simulink model "VehiclePlant"  (R2026b)
settings: Solver=ode23t  StopTime=Simulation.StopTimeSmoke.Value
undefined symbols (not defined in the file): Battery, Brake, Tire
settings Model: DataDictionary=VehicleData.sldd  Creator=Xu Dingyi  LastModifiedBy=29358
settings DebuggingCC: AlgebraicLoopMsg=error  ArtificialAlgebraicLoopMsg=error  BusObjectLabelMismatch=error

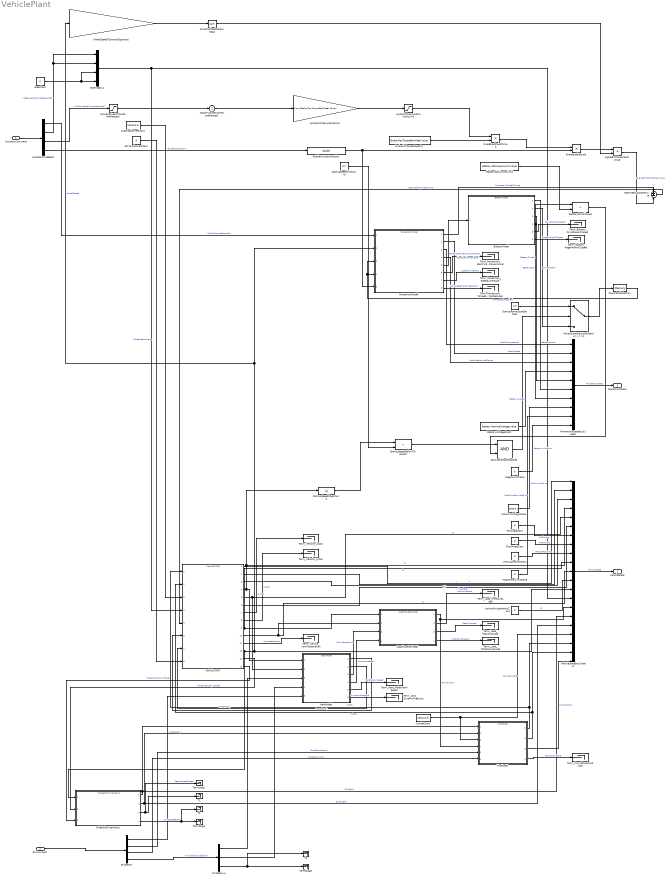
== system VehiclePlant ==
  ActuatorCommand : Inport  OutDataTypeStr=Bus: ActuatorCommandBus
  Environment : Inport  Port=2  OutDataTypeStr=Bus: EnvironmentBus
  ActuatorCmdSelect : BusSelector  OutputSignals=MotorTorqueRequest,SteeringRackAngleRequest,FrictionBrakeTorqueRequest,EnableActuation
  AeroModel : ModelReference  ModelNameDialog=AeroModel.slx  ModelReferenceVersion=2.0
  AligningMomentZero : Constant  Value=zeros(4,1)  OutDataTypeStr=double
  BatteryModel : ModelReference  ModelNameDialog=BatteryModel.slx  ModelReferenceVersion=2.0
  BatterySOCAllowed : RelationalOperator  Operator=>  OutDataTypeStr=boolean  InputSameDT=off
  BatterySOCLowerLimit : Constant  Value=Battery.SOCLowerLimit.Value  OutDataTypeStr=double
  BatteryVoltageConst : Constant  Value=Battery.NominalVoltage.Value  OutDataTypeStr=double
  BrakeEnableScale : Product  Inputs=**
  CamberZero : Constant  Value=zeros(4,1)  OutDataTypeStr=double
  EnableActuationDouble : DataTypeConversion  OutDataTypeStr=double
  EnvSelect : BusSelector  OutputSignals=AirDensity,RoadGripScale,RoadMuLimit,WindVelocityGlobal
  ExtYawMomentZero : Constant  Value=0  OutDataTypeStr=double
  FixedBiasBrakeTorque : Product  Inputs=**
  HydraulicPressureFraction : Gain  Gain=1/sum(Brake.MaxTorquePerWheel.Value)
  HydraulicPressureFractionLimit : Saturate  UpperLimit=1  LowerLimit=0
  HydraulicTorqueCapacity : Constant  Value=Brake.MaxTorquePerWheel.Value
  LoadTransferModel : ModelReference  ModelNameDialog=LoadTransferModel.slx  ModelReferenceVersion=2.1
  MotorLimitFlagsFalse : Constant  Value=false(4,1)  OutDataTypeStr=boolean
  NetWheelAppliedTorque : Sum  Inputs=+-
  NonnegativeFrictionBrakeRequest : Saturate  UpperLimit=inf(4,1)  LowerLimit=zeros(4,1)
  PitchAngleZero : Constant  Value=0  OutDataTypeStr=double
  PowerScaleMemory : Memory  InitialCondition=1
  PowerScaleStartupFallback : Switch  Threshold=0.5
  PowertrainModel : ModelReference  ModelNameDialog=PowertrainModel.slx  ModelReferenceVersion=2.0
  PowertrainStateBusCreator : BusCreator  Inputs=10  OutDataTypeStr=Bus: PowertrainStateBus
  RegenLimitFalse : Constant  Value=0  OutDataTypeStr=boolean
  RollAngleZero : Constant  Value=0  OutDataTypeStr=double
  SignedFrictionBrakeTorque : Product  Inputs=**
  SmoothWheelRotationSign : Trigonometry  Description=Continuous wheel-rotation sign approximation for stable friction braking through zero speed.  Operator=tanh
  StartupFallbackEnabled : Logic  AllPortsSameDT=off  OutDataTypeStr=boolean
  StartupPowerScaleDefault : Constant  Value=1.0  OutDataTypeStr=double
  StartupSpeedBelowThreshold : RelationalOperator  Operator=<  OutDataTypeStr=boolean  InputSameDT=off
  StartupSpeedMagnitude : Abs
  StartupSpeedThreshold : Constant  Value=0.1  OutDataTypeStr=double
  SteerZero : Constant  Value=0  OutDataTypeStr=double
  SteeringMux : Mux
  T1 : Terminator
  T2 : Terminator
  T3 : Terminator
  TermDiag1 : Terminator
  TermDiag2 : Terminator
  TermDiag3 : Terminator
  Term_Aero_DynamicPressure : Terminator
  Term_Aero_RelativeAirSpeed : Terminator
  Term_Battery_DrivePowerClipped : Terminator
  Term_Battery_RegenPowerClipped : Terminator
  Term_Load_FrontAxleLoad : Terminator
  Term_Load_RearAxleLoad : Terminator
  Term_Load_TotalNormalLoad : Terminator
  Term_Powertrain_ElectricalPowerActual : Terminator
  Term_Powertrain_SpeedLimitScale : Terminator
  Term_Powertrain_TorqueSaturationResidual : Terminator
  Term_Tire_SaturationScale : Terminator
  Term_Vehicle_UxDot : Terminator
  Term_Vehicle_UyDot : Terminator
  Term_Vehicle_YawAcceleration : Terminator
  TireModel : ModelReference  ModelNameDialog=TireModel  ModelReferenceVersion=2.0
  TotalFrictionBrakeTorqueRequest : Sum  Inputs=+
  TotalPowerLimitFalse : Constant  Value=0  OutDataTypeStr=boolean
  Vehicle7DOF : ModelReference  ModelNameDialog=Vehicle7DOF.slx  ModelReferenceVersion=2.0
  VehicleStateBusCreator : BusCreator  Inputs=21  OutDataTypeStr=Bus: VehicleStateBus
  VerticalAccelerationZero : Constant  Value=0  OutDataTypeStr=double
  VerticalPositionZero : Constant  Value=0  OutDataTypeStr=double
  WheelSlipKinematics : ModelReference  ModelNameDialog=WheelSlipKinematics.slx  ModelReferenceVersion=2.0
  WheelSpeedToSmoothSignInput : Gain  Gain=Tire.EffectiveRadius.Value/Tire.LowSpeedEpsilon.Value
  WindDemux : Demux  Outputs=3
  VehicleState : Outport  OutDataTypeStr=Bus: VehicleStateBus
  PowertrainState : Outport  Port=2  OutDataTypeStr=Bus: PowertrainStateBus
  wires:
  StartupSpeedThreshold/1 -> StartupSpeedBelowThreshold/2
  SteeringMux/1 -> VehicleStateBusCreator/14, Vehicle7DOF/4  "WheelSteerAngle"
  ActuatorCommand/1 -> ActuatorCmdSelect/1
  ActuatorCmdSelect/2 -> SteeringMux/2, SteeringMux/1  "<SteeringRackAngleRequest>"
  Environment/1 -> EnvSelect/1
  StartupSpeedMagnitude/1 -> StartupSpeedBelowThreshold/1
  SteerZero/1 -> SteeringMux/3, SteeringMux/4
  ActuatorCmdSelect/1 -> PowertrainModel/1  "<MotorTorqueRequest>"
  ActuatorCmdSelect/3 -> NonnegativeFrictionBrakeRequest/1  "<FrictionBrakeTorqueRequest>"
  ActuatorCmdSelect/4 -> EnableActuationDouble/1  "<EnableActuation>"
  TireModel/1 -> Vehicle7DOF/1, VehicleStateBusCreator/19  "TireFx"
  WheelSpeedToSmoothSignInput/1 -> SmoothWheelRotationSign/1
  LoadTransferModel/1 -> TireModel/4, VehicleStateBusCreator/15  "NormalLoad"
  NonnegativeFrictionBrakeRequest/1 -> TotalFrictionBrakeTorqueRequest/1
  AligningMomentZero/1 -> Vehicle7DOF/3
  EnvSelect/1 -> AeroModel/5  "<AirDensity>"
  ExtYawMomentZero/1 -> Vehicle7DOF/8
  StartupPowerScaleDefault/1 -> PowerScaleStartupFallback/1
  WindDemux/3 -> TermDiag3/1, T3/1
  WheelSlipKinematics/1 -> VehicleStateBusCreator/16, TireModel/1  "SlipRatio"
  WheelSlipKinematics/2 -> TireModel/2, VehicleStateBusCreator/17  "SlipAngle"
  WheelSlipKinematics/3 -> TermDiag1/1, T1/1  "RegularizedSpeed"
  WheelSlipKinematics/4 -> T2/1, TermDiag2/1  "LowSpeedBlend"
  EnableActuationDouble/1 -> BrakeEnableScale/2, PowertrainModel/5
  EnvSelect/2 -> TireModel/5  "<RoadGripScale>"
  CamberZero/1 -> VehicleStateBusCreator/18, TireModel/3  "CamberAngle"
  SmoothWheelRotationSign/1 -> SignedFrictionBrakeTorque/2
  TotalFrictionBrakeTorqueRequest/1 -> HydraulicPressureFraction/1
  Vehicle7DOF/13 -> WheelSlipKinematics/2  "WheelVelocityXWheel"
  Vehicle7DOF/9 -> LoadTransferModel/1, VehicleStateBusCreator/10  "Ax"
  Vehicle7DOF/5 -> VehicleStateBusCreator/5, AeroModel/2  "Uy"
  Vehicle7DOF/1 -> VehicleStateBusCreator/1  "X"
  Vehicle7DOF/14 -> WheelSlipKinematics/3  "WheelVelocityYWheel"
  Vehicle7DOF/10 -> VehicleStateBusCreator/11, LoadTransferModel/2  "Ay"
  Vehicle7DOF/6 -> VehicleStateBusCreator/6  "YawRate"
  Vehicle7DOF/2 -> VehicleStateBusCreator/2  "Y"
  Vehicle7DOF/11 -> Term_Vehicle_YawAcceleration/1  "YawAcceleration"
  Vehicle7DOF/7 -> Term_Vehicle_UxDot/1  "UxDot"
  Vehicle7DOF/3 -> VehicleStateBusCreator/3  "Psi"
  Vehicle7DOF/12 -> WheelSpeedToSmoothSignInput/1, PowertrainModel/2, VehicleStateBusCreator/13, WheelSlipKinematics/1  "WheelSpeed"
  Vehicle7DOF/8 -> Term_Vehicle_UyDot/1  "UyDot"
  Vehicle7DOF/4 -> VehicleStateBusCreator/4, StartupSpeedMagnitude/1, AeroModel/1  "Ux"
  WindDemux/1 -> AeroModel/3
  WindDemux/2 -> AeroModel/4
  HydraulicPressureFraction/1 -> HydraulicPressureFractionLimit/1
  AeroModel/1 -> Vehicle7DOF/6  "ForceXBody"
  AeroModel/6 -> Term_Aero_DynamicPressure/1  "DynamicPressure"
  AeroModel/4 -> LoadTransferModel/4  "DownforceRear"
  AeroModel/2 -> Vehicle7DOF/7  "ForceYBody"
  AeroModel/5 -> Term_Aero_RelativeAirSpeed/1  "RelativeAirSpeed"
  AeroModel/3 -> LoadTransferModel/3  "DownforceFront"
  HydraulicPressureFractionLimit/1 -> FixedBiasBrakeTorque/1
  HydraulicTorqueCapacity/1 -> FixedBiasBrakeTorque/2
  PowertrainModel/1 -> NetWheelAppliedTorque/1  "PowertrainWheelTorque"
  PowertrainModel/2 -> PowertrainStateBusCreator/2  "MotorSpeed"
  PowertrainModel/3 -> PowertrainStateBusCreator/1  "MotorTorqueActual"
  PowertrainModel/8 -> Term_Powertrain_TorqueSaturationResidual/1  "TorqueSaturationResidual"
  PowertrainModel/4 -> PowertrainStateBusCreator/3  "MotorMechanicalPower"
  PowertrainModel/5 -> BatteryModel/1  "ElectricalPowerUnconstrained"
  PowertrainModel/6 -> Term_Powertrain_ElectricalPowerActual/1  "ElectricalPowerActual"
  PowertrainModel/7 -> Term_Powertrain_SpeedLimitScale/1  "SpeedLimitScale"
  StartupSpeedBelowThreshold/1 -> StartupFallbackEnabled/1
  LoadTransferModel/2 -> Term_Load_FrontAxleLoad/1  "FrontAxleLoad"
  LoadTransferModel/3 -> Term_Load_RearAxleLoad/1  "RearAxleLoad"
  LoadTransferModel/4 -> Term_Load_TotalNormalLoad/1  "TotalNormalLoad"
  FixedBiasBrakeTorque/1 -> BrakeEnableScale/1
  BatterySOCLowerLimit/1 -> BatterySOCAllowed/2
  BatteryModel/1 -> PowertrainStateBusCreator/6  "BatteryPower"
  BatteryModel/2 -> PowerScaleStartupFallback/3  "PowerScale"
  BatteryModel/3 -> PowertrainStateBusCreator/5  "BatteryCurrent"
  BatteryModel/4 -> BatterySOCAllowed/1, PowertrainStateBusCreator/7  "BatterySOC"
  BatteryModel/5 -> Term_Battery_DrivePowerClipped/1  "DrivePowerClipped"
  BatteryModel/6 -> Term_Battery_RegenPowerClipped/1  "RegenPowerClipped"
  BatteryVoltageConst/1 -> PowertrainStateBusCreator/4  "BatteryVoltage"
  StartupFallbackEnabled/1 -> PowerScaleStartupFallback/2
  RegenLimitFalse/1 -> PowertrainStateBusCreator/10  "RegenLimitActive"
  MotorLimitFlagsFalse/1 -> PowertrainStateBusCreator/8  "MotorLimitActive"
  RollAngleZero/1 -> VehicleStateBusCreator/7  "RollAngle"
  PitchAngleZero/1 -> VehicleStateBusCreator/8  "PitchAngle"
  VerticalPositionZero/1 -> VehicleStateBusCreator/9  "VerticalPosition"
  TotalPowerLimitFalse/1 -> PowertrainStateBusCreator/9  "TotalPowerLimitActive"
  VerticalAccelerationZero/1 -> VehicleStateBusCreator/12  "Az"
  TireModel/2 -> Vehicle7DOF/2, VehicleStateBusCreator/20  "TireFy"
  TireModel/4 -> Term_Tire_SaturationScale/1  "SaturationScale"
  BrakeEnableScale/1 -> SignedFrictionBrakeTorque/1
  BatterySOCAllowed/1 -> StartupFallbackEnabled/2
  PowerScaleStartupFallback/1 -> PowerScaleMemory/1
  PowertrainStateBusCreator/1 -> PowertrainState/1  "PowertrainState"
  VehicleStateBusCreator/1 -> VehicleState/1  "VehicleState"
  SignedFrictionBrakeTorque/1 -> NetWheelAppliedTorque/2  "SignedFrictionBrakeTorque"
  PowerScaleMemory/1 -> PowertrainModel/4, PowertrainModel/3  "PowerScaleApplied"
  NetWheelAppliedTorque/1 -> Vehicle7DOF/5  "NetWheelAppliedTorque"
  EnvSelect/4 -> WindDemux/1  "<WindVelocityGlobal>"
  EnvSelect/3 -> TireModel/6  "<RoadMuLimit>"
  TireModel/3 -> VehicleStateBusCreator/21  "MuUtilization"
